simulink model "project"  (R2015b)
settings: Solver=FixedStepDiscrete  SolverMode=SingleTasking  StartTime=0.0  StopTime=10.0  RelTol=1e-3
libraries: shlslibv1 x68
settings Model: synDspstartup=OK  Creator=sdatta24  LastModifiedBy=agill17
settings DataIOCC: SaveOutput=off  SignalLogging=off  SaveTime=off
settings OptimizationCC: DefaultParameterBehavior=Inlined
settings DebuggingCC: AlgebraicLoopMsg=error  InheritedTsInSrcMsg=none

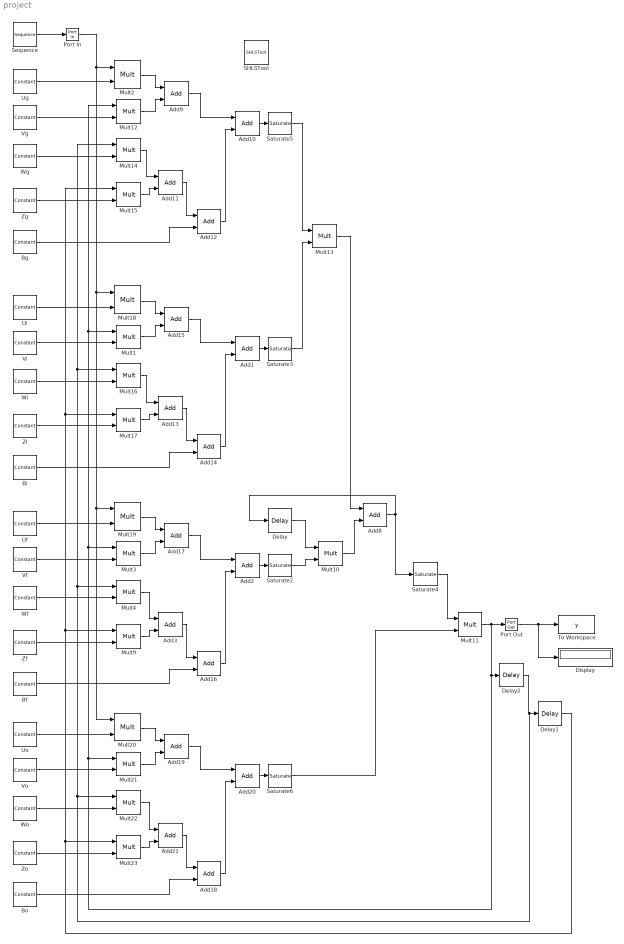
== system project ==
  Add1 : shlslibv1/Math Functions/Add  syn_add_opr=++  syn_out_f=Specify  syn_out_wl=25  syn_out_fl=7  syn_out_dt=signed  syn_out_sat=off  syn_out_rnd=Floor (Truncate)  synBlockType=primitive  synLatency=0  synBlockId=96  syn_sum_of_rows=off  syn_inh_port=off  syn_inh_st=on  syn_inh_stf=1  syn_en_pipe=off  syn_pipe_stg=syn_max_pipeline  syn_flow_ctrl=off
  Add10 : shlslibv1/Math Functions/Add  syn_add_opr=++  syn_out_f=Specify  syn_out_wl=25  syn_out_fl=7  syn_out_dt=signed  syn_out_sat=off  syn_out_rnd=Floor (Truncate)  synBlockType=primitive  synLatency=0  synBlockId=96  syn_sum_of_rows=off  syn_inh_port=off  syn_inh_st=on  syn_inh_stf=1  syn_en_pipe=off  syn_pipe_stg=syn_max_pipeline  syn_flow_ctrl=off
  Add{3,8,11..14,16,18,21} (9 alike) : shlslibv1/Math Functions/Add  syn_add_opr=++  syn_out_f=Specify  syn_out_wl=25  syn_out_fl=7  syn_out_dt=unsigned  syn_out_sat=off  syn_out_rnd=Floor (Truncate)  synBlockType=primitive  synLatency=0  synBlockId=96  syn_sum_of_rows=off  syn_inh_port=off  syn_inh_st=on  syn_inh_stf=1  syn_en_pipe=off  syn_pipe_stg=syn_max_pipeline  syn_flow_ctrl=off
  Add{9,15,17,19} (4 alike) : shlslibv1/Math Functions/Add  syn_add_opr=++  syn_out_f=Specify  syn_out_wl=25  syn_out_fl=7  syn_out_dt=unsigned  syn_out_sat=off  syn_out_rnd=Floor (Truncate)  synBlockType=primitive  synLatency=0  synBlockId=96  syn_sum_of_rows=off  syn_inh_port=off  syn_inh_st=on  syn_inh_stf=1  syn_en_pipe=on  syn_pipe_stg=2  syn_flow_ctrl=off
  Add2 : shlslibv1/Math Functions/Add  syn_add_opr=++  syn_out_f=Specify  syn_out_wl=25  syn_out_fl=7  syn_out_dt=signed  syn_out_sat=off  syn_out_rnd=Floor (Truncate)  synBlockType=primitive  synLatency=0  synBlockId=96  syn_sum_of_rows=off  syn_inh_port=off  syn_inh_st=on  syn_inh_stf=1  syn_en_pipe=off  syn_pipe_stg=syn_max_pipeline  syn_flow_ctrl=off
  Add20 : shlslibv1/Math Functions/Add  syn_add_opr=++  syn_out_f=Specify  syn_out_wl=25  syn_out_fl=7  syn_out_dt=signed  syn_out_sat=off  syn_out_rnd=Floor (Truncate)  synBlockType=primitive  synLatency=0  synBlockId=96  syn_sum_of_rows=off  syn_inh_port=off  syn_inh_st=on  syn_inh_stf=1  syn_en_pipe=on  syn_pipe_stg=4  syn_flow_ctrl=off
  Bf : shlslibv1/Sources/Constant  syn_cst_val=1  syn_cst_format=Specify  syn_cst_wl=25  syn_cst_fl=7  syn_cst_dt=unsigned  syn_cst_rnd=on  syn_cst_st=1/200e6  synBlockType=primitive  synLatency=0  synBlockId=15
  Bg : shlslibv1/Sources/Constant  syn_cst_val=1  syn_cst_format=Specify  syn_cst_wl=25  syn_cst_fl=7  syn_cst_dt=unsigned  syn_cst_rnd=on  syn_cst_st=1/200e6  synBlockType=primitive  synLatency=0  synBlockId=15
  Bi : shlslibv1/Sources/Constant  syn_cst_val=1  syn_cst_format=Specify  syn_cst_wl=25  syn_cst_fl=7  syn_cst_dt=unsigned  syn_cst_rnd=on  syn_cst_st=1/200e6  synBlockType=primitive  synLatency=0  synBlockId=15
  Bo : shlslibv1/Sources/Constant  syn_cst_val=1  syn_cst_format=Specify  syn_cst_wl=25  syn_cst_fl=7  syn_cst_dt=unsigned  syn_cst_rnd=on  syn_cst_st=1/200e6  synBlockType=primitive  synLatency=0  synBlockId=15
  Delay : shlslibv1/Memories/Delay  syn_delay_val=1  synBlockType=primitive  synLatency=1  synBlockId=104
  Delay1 : shlslibv1/Memories/Delay  syn_delay_val=9  synBlockType=primitive  synLatency=9  synBlockId=104
  Delay2 : shlslibv1/Memories/Delay  syn_delay_val=9  synBlockType=primitive  synLatency=9  synBlockId=104
  Display : Display
  Mult{1..4,9..23} (19 alike) : shlslibv1/Math Functions/Mult  syn_out_f=Specify  syn_out_wl=25  syn_out_fl=7  syn_out_dt=unsigned  syn_out_sat=off  syn_out_rnd=Floor (Truncate)  syn_inh_port=off  syn_inh_st=off  syn_inh_stf=1  syn_en_pipe=off  syn_pipe_stg=syn_max_pipeline  syn_flow_ctrl=off  synBlockType=primitive  synLatency=0  synBlockId=3  syn_opr_mode=1
  Port In : shlslibv1/Ports & Subsystems/Port In  syn_out_wl=25  syn_out_fl=7  syn_out_dt=unsigned  syn_out_st=1/200e6  syn_capture=on  syn_register=on  syn_out_sat=off  syn_out_rnd=on  synBlockType=port  synLatency=1  synBlockId=0
  Port Out : shlslibv1/Ports & Subsystems/Port Out  syn_capture=on  syn_register=on  synBlockType=port  synLatency=1  synBlockId=1
  SHLSTool : shlslibv1/SHLSTool  synBlockType=tool  syn_dsp_mode=FPGA
  Saturate2 : shlslibv1/Signal Operations/Saturate  syn_sat_mode=Constant  syn_pos_val=1  syn_neg_val=0  syn_sat_fl=7  syn_sat_rnd=on  syn_out_f=Same as Input  syn_out_wl=16  syn_out_fl=15  syn_out_dt=signed  syn_out_rnd=on  syn_pipe=on  syn_sat_ind=off  synBlockType=custom  synLatency=1
  Saturate3 : shlslibv1/Signal Operations/Saturate  syn_sat_mode=Constant  syn_pos_val=1  syn_neg_val=0  syn_sat_fl=7  syn_sat_rnd=on  syn_out_f=Same as Input  syn_out_wl=16  syn_out_fl=15  syn_out_dt=signed  syn_out_rnd=on  syn_pipe=on  syn_sat_ind=off  synBlockType=custom  synLatency=1
  Saturate4 : shlslibv1/Signal Operations/Saturate  syn_sat_mode=Constant  syn_pos_val=1  syn_neg_val=-1  syn_sat_fl=7  syn_sat_rnd=on  syn_out_f=Same as Input  syn_out_wl=16  syn_out_fl=15  syn_out_dt=signed  syn_out_rnd=on  syn_pipe=on  syn_sat_ind=off  synBlockType=custom  synLatency=1
  Saturate5 : shlslibv1/Signal Operations/Saturate  syn_sat_mode=Constant  syn_pos_val=1  syn_neg_val=-1  syn_sat_fl=7  syn_sat_rnd=on  syn_out_f=Same as Input  syn_out_wl=16  syn_out_fl=15  syn_out_dt=signed  syn_out_rnd=on  syn_pipe=on  syn_sat_ind=off  synBlockType=custom  synLatency=1
  Saturate6 : shlslibv1/Signal Operations/Saturate  syn_sat_mode=Constant  syn_pos_val=1  syn_neg_val=0  syn_sat_fl=7  syn_sat_rnd=on  syn_out_f=Same as Input  syn_out_wl=16  syn_out_fl=15  syn_out_dt=signed  syn_out_rnd=on  syn_pipe=on  syn_sat_ind=off  synBlockType=custom  synLatency=1
  Sequence : shlslibv1/Sources/Sequence  syn_seq_vec=[100 100 100 100 100 100 100 100 100 200 200 200 200 200 200 200 200 200 300 300 300 300 300 300 300 300 300 400 400 400 400 400 400 400 400 400 500 500 500 500 500 500 500 500 500 600 600 600 600 600 600 600 600 600 700 700 700 700 700 700 700 700 700 800 800 800 800 800 800 800 800 800 900 900 900 900 900 900 900 900 900]  syn_seq_wl=25  syn_seq_fl=7  syn_seq_dt=unsigned  syn_rst_port=off  syn_en_port=off  syn_seq_st=1/200e6  synBlockType=custom  synLatency=1
  To Workspace : ToWorkspace  VariableName=y  SaveFormat=Structure With Time  SampleTime=1/320e6
  Uf : shlslibv1/Sources/Constant  syn_cst_val=0  syn_cst_format=Specify  syn_cst_wl=25  syn_cst_fl=7  syn_cst_dt=unsigned  syn_cst_rnd=on  syn_cst_st=1/200e6  synBlockType=primitive  synLatency=0  synBlockId=15
  Ug : shlslibv1/Sources/Constant  syn_cst_val=1  syn_cst_format=Specify  syn_cst_wl=25  syn_cst_fl=7  syn_cst_dt=unsigned  syn_cst_rnd=on  syn_cst_st=1/200e6  synBlockType=primitive  synLatency=0  synBlockId=15
  Ui : shlslibv1/Sources/Constant  syn_cst_val=1  syn_cst_format=Specify  syn_cst_wl=25  syn_cst_fl=7  syn_cst_dt=unsigned  syn_cst_rnd=on  syn_cst_st=1/200e6  synBlockType=primitive  synLatency=0  synBlockId=15
  Uo : shlslibv1/Sources/Constant  syn_cst_val=1  syn_cst_format=Specify  syn_cst_wl=25  syn_cst_fl=7  syn_cst_dt=unsigned  syn_cst_rnd=on  syn_cst_st=1/200e6  synBlockType=primitive  synLatency=0  synBlockId=15
  Vf : shlslibv1/Sources/Constant  syn_cst_val=0  syn_cst_format=Specify  syn_cst_wl=25  syn_cst_fl=7  syn_cst_dt=unsigned  syn_cst_rnd=on  syn_cst_st=1/200e6  synBlockType=primitive  synLatency=0  synBlockId=15
  Vg : shlslibv1/Sources/Constant  syn_cst_val=1  syn_cst_format=Specify  syn_cst_wl=25  syn_cst_fl=7  syn_cst_dt=unsigned  syn_cst_rnd=on  syn_cst_st=1/200e6  synBlockType=primitive  synLatency=0  synBlockId=15
  Vi : shlslibv1/Sources/Constant  syn_cst_val=1  syn_cst_format=Specify  syn_cst_wl=25  syn_cst_fl=7  syn_cst_dt=unsigned  syn_cst_rnd=on  syn_cst_st=1/200e6  synBlockType=primitive  synLatency=0  synBlockId=15
  Vo : shlslibv1/Sources/Constant  syn_cst_val=1  syn_cst_format=Specify  syn_cst_wl=25  syn_cst_fl=7  syn_cst_dt=unsigned  syn_cst_rnd=on  syn_cst_st=1/200e6  synBlockType=primitive  synLatency=0  synBlockId=15
  Wf : shlslibv1/Sources/Constant  syn_cst_val=0  syn_cst_format=Specify  syn_cst_wl=25  syn_cst_fl=7  syn_cst_dt=unsigned  syn_cst_rnd=on  syn_cst_st=1/200e6  synBlockType=primitive  synLatency=0  synBlockId=15
  Wg : shlslibv1/Sources/Constant  syn_cst_val=1  syn_cst_format=Specify  syn_cst_wl=25  syn_cst_fl=7  syn_cst_dt=unsigned  syn_cst_rnd=on  syn_cst_st=1/200e6  synBlockType=primitive  synLatency=0  synBlockId=15
  Wi : shlslibv1/Sources/Constant  syn_cst_val=1  syn_cst_format=Specify  syn_cst_wl=25  syn_cst_fl=7  syn_cst_dt=unsigned  syn_cst_rnd=on  syn_cst_st=1/200e6  synBlockType=primitive  synLatency=0  synBlockId=15
  Wo : shlslibv1/Sources/Constant  syn_cst_val=1  syn_cst_format=Specify  syn_cst_wl=25  syn_cst_fl=7  syn_cst_dt=unsigned  syn_cst_rnd=on  syn_cst_st=1/200e6  synBlockType=primitive  synLatency=0  synBlockId=15
  Zf : shlslibv1/Sources/Constant  syn_cst_val=0  syn_cst_format=Specify  syn_cst_wl=25  syn_cst_fl=7  syn_cst_dt=unsigned  syn_cst_rnd=on  syn_cst_st=1/200e6  synBlockType=primitive  synLatency=0  synBlockId=15
  Zg : shlslibv1/Sources/Constant  syn_cst_val=1  syn_cst_format=Specify  syn_cst_wl=25  syn_cst_fl=7  syn_cst_dt=unsigned  syn_cst_rnd=on  syn_cst_st=1/200e6  synBlockType=primitive  synLatency=0  synBlockId=15
  Zi : shlslibv1/Sources/Constant  syn_cst_val=1  syn_cst_format=Specify  syn_cst_wl=25  syn_cst_fl=7  syn_cst_dt=unsigned  syn_cst_rnd=on  syn_cst_st=1/200e6  synBlockType=primitive  synLatency=0  synBlockId=15
  Zo : shlslibv1/Sources/Constant  syn_cst_val=1  syn_cst_format=Specify  syn_cst_wl=25  syn_cst_fl=7  syn_cst_dt=unsigned  syn_cst_rnd=on  syn_cst_st=1/200e6  synBlockType=primitive  synLatency=0  synBlockId=15
  wires:
  Sequence/1 -> Port In/1
  Ug/1 -> Mult2/2
  Vg/1 -> Mult12/2
  Mult2/1 -> Add9/1
  Mult12/1 -> Add9/2
  Add9/1 -> Add10/1
  Add10/1 -> Saturate5/1
  Saturate5/1 -> Mult13/1
  Wg/1 -> Mult14/2
  Zg/1 -> Mult15/2
  Mult14/1 -> Add11/1
  Mult15/1 -> Add11/2
  Add11/1 -> Add12/1
  Bg/1 -> Add12/2
  Add12/1 -> Add10/2
  Ui/1 -> Mult18/2
  Vi/1 -> Mult1/2
  Mult18/1 -> Add15/1
  Mult1/1 -> Add15/2
  Add15/1 -> Add1/1
  Add1/1 -> Saturate3/1
  Wi/1 -> Mult16/2
  Zi/1 -> Mult17/2
  Mult16/1 -> Add13/1
  Mult17/1 -> Add13/2
  Add13/1 -> Add14/1
  Bi/1 -> Add14/2
  Add14/1 -> Add1/2
  Saturate3/1 -> Mult13/2
  Uf/1 -> Mult19/2
  Vf/1 -> Mult3/2
  Mult19/1 -> Add17/1
  Mult3/1 -> Add17/2
  Add17/1 -> Add2/1
  Add2/1 -> Saturate2/1
  Wf/1 -> Mult4/2
  Zf/1 -> Mult9/2
  Mult4/1 -> Add3/1
  Mult9/1 -> Add3/2
  Add3/1 -> Add16/1
  Bf/1 -> Add16/2
  Add16/1 -> Add2/2
  Uo/1 -> Mult20/2
  Vo/1 -> Mult21/2
  Mult20/1 -> Add19/1
  Mult21/1 -> Add19/2
  Add19/1 -> Add20/1
  Add20/1 -> Saturate6/1
  Wo/1 -> Mult22/2
  Zo/1 -> Mult23/2
  Mult22/1 -> Add21/1
  Mult23/1 -> Add21/2
  Add21/1 -> Add18/1
  Bo/1 -> Add18/2
  Add18/1 -> Add20/2
  Mult11/1 -> Mult21/1, Mult3/1, Mult1/1, Mult12/1, Delay2/1, Port Out/1
  Delay/1 -> Mult10/1
  Mult10/1 -> Add8/2
  Add8/1 -> Delay/1, Saturate4/1
  Port Out/1 -> Display/1, To Workspace/1
  Saturate4/1 -> Mult11/1
  Saturate2/1 -> Mult10/2
  Mult13/1 -> Add8/1
  Saturate6/1 -> Mult11/2
  Delay2/1 -> Mult22/1, Mult4/1, Mult16/1, Mult14/1, Delay1/1
  Delay1/1 -> Mult23/1, Mult9/1, Mult17/1, Mult15/1
  Port In/1 -> Mult19/1, Mult20/1, Mult18/1, Mult2/1
